simulink model "tqdtqr_rebuild_V3"  (R2021b)
settings: Solver=VariableStepAuto  StartTime=0.0  StopTime=10.0  RelTol=1e-3
undefined symbols (not defined in the file): ATQD_AfterTqMinGain_X_Deg, ATQD_APSCreepBaseTqD_X_kph, ATQD_APSCreepBaseTqD_Y_Deg, ATQD_APSCreepBaseTqR_X_kph, ATQD_APSCreepBaseTqR_Y_Deg, ATQD_APSCreepIterm_X_kph, ATQD_APSCreepIterm_Y_kph, ATQD_APSCreepPterm_X_kph, ATQD_APSCreepPterm_Y_kph, ATQD_APSDecReq_X_kph, ATQD_APSDecReq_Y_mps2, ATQD_APSDecReqCMD_X_kph, ATQD_APSDecReqTs_X_pct, ATQD_APSDecTimeGain_X_Deg, ATQD_APSDecTimeGain_Y_s, ATQD_APSReqLowSpd_X_Deg, ATQD_AutoHoldReleaseBPS_X_Deg, ATQD_AWDLoadTrqnsGain_X_kg, ATQD_AWDLoadTrqnsGain_Y_pct, ATQD_BOSEnBPSPosn_X_kph, ATQD_BOSMap_X_rpm, ATQD_BOSMap_Y_pct, ATQD_CreepBaseTqD_X_kph, ATQD_CreepBaseTqD_Y_Deg, ATQD_CreepBaseTqR_X_kph, ATQD_CreepBaseTqR_Y_Deg, ATQD_CreepBPSDisPosn_X_Deg, ATQD_CreepBPSDisPosnR_X_Deg, ATQD_CreepBPSEnPosn_X_Deg, ATQD_CreepBPSEnPosnR_X_Deg, ATQD_CreepDeltaTq_X_kph, ATQD_CreepIterm_X_kph, ATQD_CreepIterm_Y_kph, ATQD_CreepItermMaxLimit_X_pct, ATQD_CreepPreloadTime_X_kph, ATQD_CreepPreloadTq_X_kph, ATQD_CreepPreloadTq_Y_s, ATQD_CreepProtTq_X_Deg, ATQD_CreepPterm_X_kph, ATQD_CreepPterm_Y_kph, ATQD_CreepRrTqSpRat_X_rpm, ATQD_CreepRrTqSpRat_Y_Nm, ATQD_CreepTargetSpdD_X_pct, ATQD_CreepTargetSpdR_X_pct, ATQD_CreepUpLimitTq_X_rpm, ATQD_DecIneOPDHoldEnDelay_X_Deg, ATQD_DecIneOPDHoldEnDelay_Y_bar, ATQD_ECOTqMapD_X_rpm, ATQD_ECOTqMapD_Y_pct, ATQD_EMTqMapD_X_rpm, ATQD_EMTqMapD_Y_pct, ATQD_EOPDTqMapDCon_X_rpm, ATQD_EOPDTqMapDCon_Y_Deg, ATQD_EstInitVehWeight_X_c, ATQD_FAfterTqCMDGain_X_rpm, ATQD_FAfterTqCMDGain_Y_pct, ATQD_ForceLowSpd_X_Deg, ATQD_ForcePLimitSpd_X_Deg, ATQD_FrLossMAPLowV_X_rpm, ATQD_FrLossMAPLowV_Y_Nm ... (+949)
libraries: simulink x235, hcu_lib x208, tqr x63, tqd x6
(part 2 of 37)

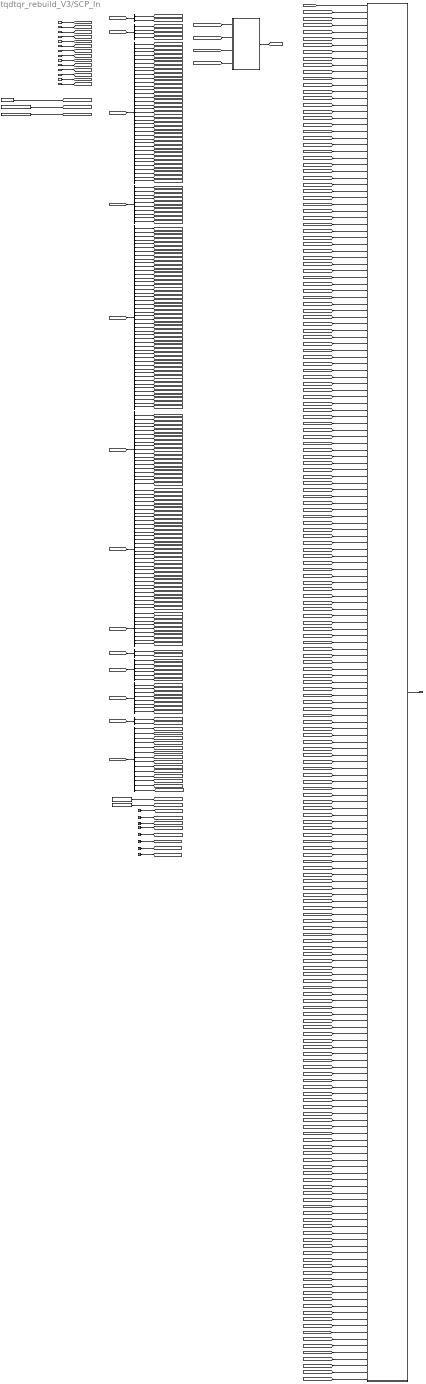
== system tqdtqr_rebuild_V3/SCP_In ==
  task_time_s : Inport
  BDHP_outputs : Inport  Port=2
  BPMM_outputs : Inport  Port=3
  BINP_CAN1_outputs : Inport  Port=4
  BINP_CAN2_outputs : Inport  Port=5
  BINP_CAN3_outputs : Inport  Port=6
  BINP_CAN4_outputs : Inport  Port=7
  BVMC_outputs : Inport  Port=8
  BINP_GPIO_outputs : Inport  Port=9
  BBCM_outputs : Inport  Port=10
  BINP_CAN6_outputs : Inport  Port=11
  BINP_SYS_outputs : Inport  Port=12
  BINP_APM_outputs : Inport  Port=13
  BDDM_outputs : Inport  Port=14
  Bus Selector : BusSelector  OutputSignals=VINP_IVIPWModeReq_enum,VINP_IVICreepSWReq_flg,VINP_RollModeSWCmd_enum,VINP_IVIPwrLockSW_enum,VINP_IVIISAOffsetSpd_enum,VINP_Distanceunit_flg,VINP_SmartEcoModeSW_flg,VINP_IVISnowModeCmd_flg,VINP_IVIACCAdaptiveSta_flg,VINP_IVITrailerModeSWSta_flg
  Bus Selector1 : BusSelector  OutputSignals=VDHP_ActAPSPosn_pct,VDHP_LowIdleAccPedal_flg
  Bus Selector10 : BusSelector  OutputSignals=VBCM_BrakeLamp_flg,VBCM_UserNow_enum
  Bus Selector11 : BusSelector  OutputSignals=VINP_FlashRegenMode_enum,VINP_VehicleType_enum,VINP_SWCType_enum,VINP_DIDGetDynoMode_flg,VINP_CAN1BusOff_flg,VINP_CAN1BusError_flg,VINP_CAN2BusOff_flg,VINP_CAN2BusError_flg
  Bus Selector12 : BusSelector  OutputSignals=VINP_CAASSta_enum,VINP_APSStaSystem_enum
  Bus Selector15 : BusSelector  OutputSignals=VDDM_VCURAPSErrLv2_flg,VDDM_VCURAPSErrLv3_flg,VDDM_EPBSigErrCFS_flg,VDDM_EPB1Err_flg,VDDM_ESC1Err_flg,VDDM_ESC5Err_flg,VDDM_LimpHomeAct_flg,VDDM_VehMalfunLevel_enum,VDDM_Shifter1Err_flg,VDDM_ShifterSigErrCFS_flg,VDDM_MCUF1Err_flg,VDDM_MCUR1Err_flg,VDDM_RegenErrCFS_flg,VDDM_4D2CErr_flg
  Bus Selector2 : BusSelector  OutputSignals=VINP_VehSpeed_kph,VINP_BrkSwSta_flg,VINP_BrkSwV_flg,VINP_BrkPedalPos_pct,VINP_BrkPedalPosSta_flg,VINP_FrPTCSActive_flg,VINP_RrPTCSActive_flg,VINP_FrntAxlTrqReqDrv_Nm,VINP_RearAxlTrqReqDrv_Nm,VINP_FrRBCActive_flg,VINP_RrRBCActive_flg,VINP_FrntAxlTrqReqBrk_Nm,VINP_RearAxlTrqReqBrk_Nm,VINP_CrashOutputSts_enum,VINP_LongAccel_Gps,VINP_EPBCarWashMode_flg,VINP_EPBErrSta_enum,VINP_EPBSta_enum,VINP_DOASta_flg,VINP_GRADE_Deg,VINP_HSAActive_flg,VINP_DriverSeatBeltCmd_flg,VINP_AVHActive_flg,VINP_PsngrSeatBeltCmd_flg,VINP_RDriverSeatBeltCmd_flg,VINP_RCenterSeatBeltCmd_flg,VINP_RPsngrSeatBeltCmd_flg,VINP_YawRate_degps,VINP_SASAngle_Deg,VINP_ESCActive_flg,VINP_ABSActive_flg,VINP_LFRawWhlSpeed_kph,VINP_LRRawWhlSpeed_kph,VINP_RFRawWhlSpeed_kph,VINP_RRRawWhlSpeed_kph,VINP_ESCOFFStatus_enum,VINP_MCPressure_bar
  Bus Selector3 : BusSelector  OutputSignals=VINP_BrakeSWGPIO_flg,VINP_CrashSignalGPIO_flg,VINP_DrDoorSW_flg,VINP_SeatSW_flg,VINP_HoodSW_flg,VINP_TailgateSW_flg,VINP_PsDoorSW_flg,VINP_RRDoorSW_flg,VINP_RLDoorSW_flg
  Bus Selector4 : BusSelector  OutputSignals=VINP_ShifterHandleCmd_enum,VINP_HVBPwrAvailDchrg_kW,VINP_HVBPwrAvailChrg_kW,VINP_HVBattErr_flg,VINP_DCDCFaultSta_enum,VINP_ChrgPlugSta_enum,VINP_HVBattSOC_pct,VINP_HVBattSOCDis_pct,VINP_HVBMTempMax_C,VINP_HVBMTempMin_C,VINP_ShifterFailsta_enum,VINP_CANMsgValidMCUNR1_flg,VINP_FrEDURotateDirctionNidec_enum,VINP_FrEDURotateDirction_enum,VINP_RrEDURotateDirctionNidec_enum,VINP_RrEDURotateDirction_enum,VINP_FrTMSpdNidec_rpm,VINP_FrTMSpd_rpm,VINP_RrTMSpdNidec_rpm,VINP_RrTMSpd_rpm,VINP_FrRegenAvailTqNidec_Nm,VINP_FrRegenAvailTq_Nm,VINP_RrRegenAvailTqNidec_Nm,VINP_RrRegenAvailTq_Nm,VINP_FrEDURealTMTqNidec_Nm,VINP_FrEDURealTMTq_Nm,VINP_RrEDURealTMTqNidec_Nm,VINP_RrEDURealTMTq_Nm,VINP_FrMotorAvailTqNidec_Nm,VINP_FrMotorAvailTq_Nm,VINP_RrMotorAvailTqNidec_Nm,VINP_RrMotorAvailTq_Nm,VINP_MCUWarnFNidec_enum,VINP_MCUWarnF_enum,VINP_MCUWarnRNidec_enum,VINP_MCUWarnR_enum,VINP_FrMCUDCBusVoltNidec_V,VINP_FrMCUDCBusVolt_V,VINP_RrMCUDCBusVoltNidec_V,VINP_RrMCUDCBusVolt_V,VINP_FrMCUTempNidec_C,VINP_FrMCUTemp_C,VINP_FrTMTempNidec_C,VINP_FrTMTemp_C,VINP_RrMCUTempNidec_C,VINP_RrMCUTemp_C,VINP_RrTMTempNidec_C,VINP_RrTMTemp_C
  Bus Selector5 : BusSelector  OutputSignals=VVMC_ADASForceIdle_flg,VVMC_ACCRequiredAccel_mps2,VVMC_ACCVehHoldReq_flg,VVMC_ADASActive_flg,VVMC_ADASWhlTqReq_Nm,VVMC_CruzActive_flg,VVMC_CruzWhlTqReq_Nm,VVMC_MSAActive_flg,VVMC_MSAWhlTqReq_Nm,VVMC_APSActive_flg,VVMC_APSSpeedCMD_kph,VVMC_APSShiftPosnReq_enum,VVMC_ACCPedalOvrd_flg,VVMC_LongAcc_Gps,VVMC_ActMaxSlideRate_pct,VVMC_EstSlope_Deg,VVMC_APSReq_enum,VVMC_RWDRDCActive_enum,VVMC_ActLRSlideRate_pct,VVMC_ActRRSlideRate_pct,VVMC_ActStESCYaw_Dps,VVMC_CCCtrlSta_enum,VVMC_MSACtrlSta_enum,VVMC_LVDAACCStatusInformation_flg,VVMC_ACCObjDist_m,VVMC_MeterIndSpeed_raw32,VVMC_RearTqRatio_rat,VVMC_CalibratedGyroY_Dps,VVMC_CAASActive_flg,VVMC_SetACCDisableAPS_flg,VVMC_CCPedalOvrd_flg,VVMC_MSAWhlTqActive_flg
  Bus Selector6 : BusSelector  OutputSignals=VINP_SWCResUpSta_flg,VINP_SWCSetdownSta_flg,VINP_SWCACCSta_flg,VINP_SWCCANCELSta_flg,VINP_SWC2LScrollUpSta_flg,VINP_SWC2LScrollDownSta_flg,VINP_SWC2LScrollPressSta_flg,VINP_SWC2LADASSta_flg,VINP_SWC2RScrollPressSta_flg,VINP_SWC2RScrollUpSta_flg,VINP_SWC2RScrollDownSta_flg,VINP_SWC2LDriveModeSta_flg,VINP_SWC2RRightSta_flg,VINP_SWC2RLeftSta_flg,VINP_SWC2RCustomizeSta_flg,VINP_SWC2LRegenUpSta_flg,VINP_SWC2RRegenDownSta_flg,VINP_SWCRegenDown_flg,VINP_SWCRegenUp_flg
  Bus Selector7 : BusSelector  OutputSignals=VPMM_PowerSta_enum,VPMM_DrivetrainSelect_enum,VPMM_SysPowerMode_enum,VPMM_DrSeatSta_enum
  Bus Selector9 : BusSelector  OutputSignals=VINP_ADASISASta_enum,VINP_ADASVehSpdLim_enum,VINP_ADASACCSta_enum,VINP_ADASSLIFSpdLim_enum,VINP_ADASAEBSta_enum,VINP_ACCVehHoldReq_flg
  Constant : Constant  Value=ZERO_INT
  Constant1 : Constant  Value=KTQD_BCMUserNowSetting_enum
  Constant12 : Constant  Value=KTQD_DIDNVHPedalLim_flg
  Constant2 : Constant  Value=KTQD_IVIRockModeCmd_flg
  Constant3 : Constant  Value=KTQD_DIDExhibitMode_enum
  Ground{,1..7} (8 alike) : Ground
  Input Signal : Subsystem
  Invalid Condition : Subsystem
  BSCPIn_outputs : Outport
  wires:
  task_time_s/1 -> [task_time_s]
  BDHP_outputs/1 -> [BDHP_outputs]
  BPMM_outputs/1 -> [BPMM_outputs]
  BINP_CAN1_outputs/1 -> [BINP_CAN1_outputs]
  BINP_CAN2_outputs/1 -> [BINP_CAN2_outputs]
  BINP_CAN3_outputs/1 -> [BINP_CAN3_outputs]
  BINP_CAN4_outputs/1 -> [BINP_CAN4_outputs]
  BVMC_outputs/1 -> [BVMC_outputs]
  BINP_GPIO_outputs/1 -> [BINP_GPIO_outputs]
  BBCM_outputs/1 -> [BBCM_outputs]
  BINP_CAN6_outputs/1 -> [BINP_CAN6_outputs]
  BINP_SYS_outputs/1 -> [BINP_SYS_outputs]
  BINP_APM_outputs/1 -> [BINP_APM_outputs]
  BDDM_outputs/1 -> [BDDM_outputs]
  [BDHP_outputs] -> Bus Selector1/1
  Bus Selector1/1 -> [VDHP_ActAPSPosn_pct]  "<VDHP_ActAPSPosn_pct>"
  Bus Selector1/2 -> [VDHP_LowIdleAccPedal_flg]  "<VDHP_LowIdleAccPedal_flg>"
  [BPMM_outputs] -> Bus Selector7/1
  Bus Selector7/1 -> [VPMM_PowerSta_enum]  "<VPMM_PowerSta_enum>"
  Bus Selector7/2 -> [VPMM_DrivetrainSelect_enum]  "<VPMM_DrivetrainSelect_enum>"
  Bus Selector7/3 -> [VPMM_SysPowerMode_enum]  "<VPMM_SysPowerMode_enum>"
  [BINP_CAN1_outputs] -> Bus Selector2/1
  Bus Selector2/1 -> [VINP_VehSpeed_kph]  "<VINP_VehSpeed_kph>"
  Bus Selector2/2 -> [VINP_BrkSwSta_flg]  "<VINP_BrkSwSta_flg>"
  Bus Selector2/3 -> [VINP_BrkSwV_flg]  "<VINP_BrkSwV_flg>"
  Bus Selector2/4 -> [VINP_BrkPedalPos_pct]  "<VINP_BrkPedalPos_pct>"
  Bus Selector2/5 -> [VINP_BrkPedalPosSta_flg]  "<VINP_BrkPedalPosSta_flg>"
  Bus Selector2/6 -> [VINP_FrPTCSActive_flg]  "<VINP_FrPTCSActive_flg>"
  Bus Selector2/7 -> [VINP_RrPTCSActive_flg]  "<VINP_RrPTCSActive_flg>"
  Bus Selector2/8 -> [VINP_FrntAxlTrqReqDrv_Nm]  "<VINP_FrntAxlTrqReqDrv_Nm>"
  Bus Selector2/9 -> [VINP_RearAxlTrqReqDrv_Nm]  "<VINP_RearAxlTrqReqDrv_Nm>"
  Bus Selector2/10 -> [VINP_FrRBCActive_flg]  "<VINP_FrRBCActive_flg>"
  Bus Selector2/11 -> [VINP_RrRBCActive_flg]  "<VINP_RrRBCActive_flg>"
  Bus Selector2/12 -> [VINP_FrntAxlTrqReqBrk_Nm]  "<VINP_FrntAxlTrqReqBrk_Nm>"
  Bus Selector2/13 -> [VINP_RearAxlTrqReqBrk_Nm]  "<VINP_RearAxlTrqReqBrk_Nm>"
  Bus Selector2/14 -> [VINP_CrashOutputSts_enum]  "<VINP_CrashOutputSts_enum>"
  Bus Selector2/15 -> [VINP_LongAccel_Gps]  "<VINP_LongAccel_Gps>"
  Bus Selector2/16 -> [VINP_EPBCarWashMode_flg]  "<VINP_EPBCarWashMode_flg>"
  Bus Selector2/17 -> [VINP_EPBErrSta_enum]  "<VINP_EPBErrSta_enum>"
  Bus Selector2/18 -> [VINP_EPBSta_enum]  "<VINP_EPBSta_enum>"
  Bus Selector2/19 -> [VINP_DOASta_flg]  "<VINP_DOASta_flg>"
  Bus Selector2/20 -> [VINP_GRADE_Deg]  "<VINP_GRADE_Deg>"
  Bus Selector2/21 -> [VINP_HSAActive_flg]  "<VINP_HSAActive_flg>"
  Bus Selector2/22 -> [VINP_DriverSeatBeltCmd_flg]  "<VINP_DriverSeatBeltCmd_flg>"
  Bus Selector2/23 -> [VINP_AVHActive_flg]  "<VINP_AVHActive_flg>"
  Bus Selector2/24 -> [VINP_PsngrSeatBeltCmd_flg]  "<VINP_PsngrSeatBeltCmd_flg>"
  Bus Selector2/25 -> [VINP_RDriverSeatBeltCmd_flg]  "<VINP_RDriverSeatBeltCmd_flg>"
  Bus Selector2/26 -> [VINP_RCenterSeatBeltCmd_flg]  "<VINP_RCenterSeatBeltCmd_flg>"
  Bus Selector2/27 -> [VINP_RPsngrSeatBeltCmd_flg]  "<VINP_RPsngrSeatBeltCmd_flg>"
  Bus Selector2/28 -> [VINP_YawRate_degps]  "<VINP_YawRate_degps>"
  Bus Selector2/29 -> [VINP_SASAngle_Deg]  "<VINP_SASAngle_Deg>"
  Bus Selector2/30 -> [VINP_ESCActive_flg]  "<VINP_ESCActive_flg>"
  Bus Selector2/31 -> [VINP_ABSActive_flg]  "<VINP_ABSActive_flg>"
  Bus Selector2/32 -> [VINP_LFRawWhlSpeed_kph]  "<VINP_LFRawWhlSpeed_kph>"
  Bus Selector2/33 -> [VINP_LRRawWhlSpeed_kph]  "<VINP_LRRawWhlSpeed_kph>"
  Bus Selector2/34 -> [VINP_RFRawWhlSpeed_kph]  "<VINP_RFRawWhlSpeed_kph>"
  Bus Selector2/35 -> [VINP_RRRawWhlSpeed_kph]  "<VINP_RRRawWhlSpeed_kph>"
  Bus Selector2/36 -> [VINP_ESCOFFStatus_enum]  "<VINP_ESCOFFStatus_enum>"
  [BINP_CAN2_outputs] -> Bus Selector/1
  Bus Selector/1 -> [VINP_IVIPWModeReq_enum]  "<VINP_IVIPWModeReq_enum>"
  Bus Selector/2 -> [VINP_IVICreepSWReq_flg]  "<VINP_IVICreepSWReq_flg>"
  Bus Selector/3 -> [VINP_RollModeSWCmd_enum]  "<VINP_RollModeSWCmd_enum>"
  Bus Selector/4 -> [VINP_IVIPwrLockSW_enum]  "<VINP_IVIPwrLockSW_enum>"
  Bus Selector/5 -> [VINP_IVIISAOffsetSpd_enum]  "<VINP_IVIISAOffsetSpd_enum>"
  Bus Selector/6 -> [VINP_Distanceunit_flg]  "<VINP_Distanceunit_flg>"
  Bus Selector/7 -> [VINP_SmartEcoModeSW_flg]  "<VINP_SmartEcoModeSW_flg>"
  Bus Selector/8 -> [VINP_IVISnowModeCmd_flg]  "<VINP_IVISnowModeCmd_flg>"
  Bus Selector/9 -> [VINP_IVIACCAdaptiveSta_flg]  "<VINP_IVIACCAdaptiveSta_flg>"
  Bus Selector/10 -> [VINP_IVITrailerModeSWSta_flg]  "<VINP_IVITrailerModeSWSta_flg>"
  [BINP_CAN3_outputs] -> Bus Selector4/1
  Bus Selector4/1 -> [VINP_ShifterHandleCmd_enum]  "<VINP_ShifterHandleCmd_enum>"
  Bus Selector4/2 -> [VINP_HVBPwrAvailDchrg_kW]  "<VINP_HVBPwrAvailDchrg_kW>"
  Bus Selector4/3 -> [VINP_HVBPwrAvailChrg_kW]  "<VINP_HVBPwrAvailChrg_kW>"
  Bus Selector4/4 -> [VINP_HVBattErr_flg]  "<VINP_HVBattErr_flg>"
  Bus Selector4/5 -> [VINP_DCDCFaultSta_enum]  "<VINP_DCDCFaultSta_enum>"
  Bus Selector4/6 -> [VINP_ChrgPlugSta_enum]  "<VINP_ChrgPlugSta_enum>"
  Bus Selector4/7 -> [VINP_HVBattSOC_pct]  "<VINP_HVBattSOC_pct>"
  Bus Selector4/8 -> [VINP_HVBattSOCDis_pct]  "<VINP_HVBattSOCDis_pct>"
  Bus Selector4/9 -> [VINP_HVBMTempMax_C]  "<VINP_HVBMTempMax_C>"
  Bus Selector4/10 -> [VINP_HVBMTempMin_C]  "<VINP_HVBMTempMin_C>"
  Bus Selector4/11 -> [VINP_ShifterFailsta_enum]  "<VINP_ShifterFailsta_enum>"
  Bus Selector4/12 -> [VINP_CANMsgValidMCUNR1_flg]  "<VINP_CANMsgValidMCUNR1_flg>"
  Bus Selector4/13 -> [VINP_FrEDURotateDirctionNidec_enum]  "<VINP_FrEDURotateDirctionNidec_enum>"
  Bus Selector4/14 -> [VINP_FrEDURotateDirction_enum]  "<VINP_FrEDURotateDirction_enum>"
  Bus Selector4/15 -> [VINP_RrEDURotateDirctionNidec_enum]  "<VINP_RrEDURotateDirctionNidec_enum>"
  Bus Selector4/16 -> [VINP_RrEDURotateDirction_enum]  "<VINP_RrEDURotateDirction_enum>"
  Bus Selector4/17 -> [VINP_FrTMSpdNidec_rpm]  "<VINP_FrTMSpdNidec_rpm>"
  Bus Selector4/18 -> [VINP_FrTMSpd_rpm]  "<VINP_FrTMSpd_rpm>"
  Bus Selector4/19 -> [VINP_RrTMSpdNidec_rpm]  "<VINP_RrTMSpdNidec_rpm>"
  Bus Selector4/20 -> [VINP_RrTMSpd_rpm]  "<VINP_RrTMSpd_rpm>"
  Bus Selector4/21 -> [VINP_FrRegenAvailTqNidec_Nm]  "<VINP_FrRegenAvailTqNidec_Nm>"
  Bus Selector4/22 -> [VINP_FrRegenAvailTq_Nm]  "<VINP_FrRegenAvailTq_Nm>"
  Bus Selector4/23 -> [VINP_RrRegenAvailTqNidec_Nm]  "<VINP_RrRegenAvailTqNidec_Nm>"
  Bus Selector4/24 -> [VINP_RrRegenAvailTq_Nm]  "<VINP_RrRegenAvailTq_Nm>"
  Bus Selector4/25 -> [VINP_FrEDURealTMTqNidec_Nm]  "<VINP_FrEDURealTMTqNidec_Nm>"
  Bus Selector4/26 -> [VINP_FrEDURealTMTq_Nm]  "<VINP_FrEDURealTMTq_Nm>"
  Bus Selector4/27 -> [VINP_RrEDURealTMTqNidec_Nm]  "<VINP_RrEDURealTMTqNidec_Nm>"
  Bus Selector4/28 -> [VINP_RrEDURealTMTq_Nm]  "<VINP_RrEDURealTMTq_Nm>"
  Bus Selector4/29 -> [VINP_FrMotorAvailTqNidec_Nm]  "<VINP_FrMotorAvailTqNidec_Nm>"
  Bus Selector4/30 -> [VINP_FrMotorAvailTq_Nm]  "<VINP_FrMotorAvailTq_Nm>"
  Bus Selector4/31 -> [VINP_RrMotorAvailTqNidec_Nm]  "<VINP_RrMotorAvailTqNidec_Nm>"
  Bus Selector4/32 -> [VINP_RrMotorAvailTq_Nm]  "<VINP_RrMotorAvailTq_Nm>"
  Bus Selector4/33 -> [VINP_MCUWarnFNidec_enum]  "<VINP_MCUWarnFNidec_enum>"
  Bus Selector4/34 -> [VINP_MCUWarnF_enum]  "<VINP_MCUWarnF_enum>"
  Bus Selector4/35 -> [VINP_MCUWarnRNidec_enum]  "<VINP_MCUWarnRNidec_enum>"
  Bus Selector4/36 -> [VINP_MCUWarnR_enum]  "<VINP_MCUWarnR_enum>"
  Bus Selector4/37 -> [VINP_FrMCUDCBusVoltNidec_V]  "<VINP_FrMCUDCBusVoltNidec_V>"
  Bus Selector4/38 -> [VINP_FrMCUDCBusVolt_V]  "<VINP_FrMCUDCBusVolt_V>"
  Bus Selector4/39 -> [VINP_RrMCUDCBusVoltNidec_V]  "<VINP_RrMCUDCBusVoltNidec_V>"
  Bus Selector4/40 -> [VINP_RrMCUDCBusVolt_V]  "<VINP_RrMCUDCBusVolt_V>"
  Bus Selector4/41 -> [VINP_FrMCUTempNidec_C]  "<VINP_FrMCUTempNidec_C>"
  Bus Selector4/42 -> [VINP_FrMCUTemp_C]  "<VINP_FrMCUTemp_C>"
  Bus Selector4/43 -> [VINP_FrTMTempNidec_C]  "<VINP_FrTMTempNidec_C>"
  Bus Selector4/44 -> [VINP_FrTMTemp_C]  "<VINP_FrTMTemp_C>"
  Bus Selector4/45 -> [VINP_RrMCUTempNidec_C]  "<VINP_RrMCUTempNidec_C>"
  Bus Selector4/46 -> [VINP_RrMCUTemp_C]  "<VINP_RrMCUTemp_C>"
  Bus Selector4/47 -> [VINP_RrTMTempNidec_C]  "<VINP_RrTMTempNidec_C>"
  Bus Selector4/48 -> [VINP_RrTMTemp_C]  "<VINP_RrTMTemp_C>"
  [BINP_CAN4_outputs] -> Bus Selector6/1
  Bus Selector6/1 -> [VINP_SWCResUpSta_flg]  "<VINP_SWCResUpSta_flg>"
  Bus Selector6/2 -> [VINP_SWCSetdownSta_flg]  "<VINP_SWCSetdownSta_flg>"
  Bus Selector6/3 -> [VINP_SWCACCSta_flg]  "<VINP_SWCACCSta_flg>"
  Bus Selector6/4 -> [VINP_SWCCANCELSta_flg]  "<VINP_SWCCANCELSta_flg>"
  Bus Selector6/5 -> [VINP_SWC2LScrollUpSta_flg]  "<VINP_SWC2LScrollUpSta_flg>"
  Bus Selector6/6 -> [VINP_SWC2LScrollDownSta_flg]  "<VINP_SWC2LScrollDownSta_flg>"
  Bus Selector6/7 -> [VINP_SWC2LScrollPressSta_flg]  "<VINP_SWC2LScrollPressSta_flg>"
  Bus Selector6/8 -> [VINP_SWC2LADASSta_flg]  "<VINP_SWC2LADASSta_flg>"
  Bus Selector6/9 -> [VINP_SWC2RScrollPressSta_flg]  "<VINP_SWC2RScrollPressSta_flg>"
  Bus Selector6/10 -> [VINP_SWC2RScrollUpSta_flg]  "<VINP_SWC2RScrollUpSta_flg>"
  Bus Selector6/11 -> [VINP_SWC2RScrollDownSta_flg]  "<VINP_SWC2RScrollDownSta_flg>"
  Bus Selector6/12 -> [VINP_SWC2LDriveModeSta_flg]  "<VINP_SWC2LDriveModeSta_flg>"
  Bus Selector6/13 -> [VINP_SWC2RRightSta_flg]  "<VINP_SWC2RRightSta_flg>"
  Bus Selector6/14 -> [VINP_SWC2RLeftSta_flg]  "<VINP_SWC2RLeftSta_flg>"
  Bus Selector6/15 -> [VINP_SWC2RCustomizeSta_flg]  "<VINP_SWC2RCustomizeSta_flg>"
  Bus Selector6/16 -> [VINP_SWC2LRegenUpSta_flg]  "<VINP_SWC2LRegenUpSta_flg>"
  Bus Selector6/17 -> [VINP_SWC2RRegenDownSta_flg]  "<VINP_SWC2RRegenDownSta_flg>"
  Bus Selector6/18 -> [VINP_SWCRegenDown_flg]  "<VINP_SWCRegenDown_flg>"
  Bus Selector6/19 -> [VINP_SWCRegenUp_flg]  "<VINP_SWCRegenUp_flg>"
  [BVMC_outputs] -> Bus Selector5/1
  Bus Selector5/1 -> [VVMC_ADASForceIdle_flg]  "<VVMC_ADASForceIdle_flg>"
  Bus Selector5/2 -> [VVMC_ACCRequiredAccel_mps2]  "<VVMC_ACCRequiredAccel_mps2>"
  Bus Selector5/3 -> [VVMC_ACCVehHoldReq_flg]  "<VVMC_ACCVehHoldReq_flg>"
  Bus Selector5/4 -> [VVMC_ADASActive_flg]  "<VVMC_ADASActive_flg>"
  Bus Selector5/5 -> [VVMC_ADASWhlTqReq_Nm]  "<VVMC_ADASWhlTqReq_Nm>"
  Bus Selector5/6 -> [VVMC_CruzActive_flg]  "<VVMC_CruzActive_flg>"
  Bus Selector5/7 -> [VVMC_CruzWhlTqReq_Nm]  "<VVMC_CruzWhlTqReq_Nm>"
  Bus Selector5/8 -> [VVMC_MSAActive_flg]  "<VVMC_MSAActive_flg>"
  Bus Selector5/9 -> [VVMC_MSAWhlTqReq_Nm]  "<VVMC_MSAWhlTqReq_Nm>"
  Bus Selector5/10 -> [VVMC_APSActive_flg]  "<VVMC_APSActive_flg>"
  Bus Selector5/11 -> [VVMC_APSSpeedCMD_kph]  "<VVMC_APSSpeedCMD_kph>"
  Bus Selector5/12 -> [VVMC_APSShiftPosnReq_enum]  "<VVMC_APSShiftPosnReq_enum>"
  Bus Selector5/13 -> [VVMC_ACCPedalOvrd_flg]  "<VVMC_ACCPedalOvrd_flg>"
  Bus Selector5/14 -> [VVMC_LongAcc_Gps]  "<VVMC_LongAcc_Gps>"
  Bus Selector5/15 -> [VVMC_ActMaxSlideRate_pct]  "<VVMC_ActMaxSlideRate_pct>"
  Bus Selector5/16 -> [VVMC_EstSlope_Deg]  "<VVMC_EstSlope_Deg>"
  Bus Selector5/17 -> [VVMC_APSReq_enum]  "<VVMC_APSReq_enum>"
  Bus Selector5/18 -> [VVMC_RWDRDCActive_enum]  "<VVMC_RWDRDCActive_enum>"
  Bus Selector5/19 -> [VVMC_ActLRSlideRate_pct]  "<VVMC_ActLRSlideRate_pct>"
  Bus Selector5/20 -> [VVMC_ActRRSlideRate_pct]  "<VVMC_ActRRSlideRate_pct>"
  Bus Selector5/21 -> [VVMC_ActStESCYaw_Dps]  "<VVMC_ActStESCYaw_Dps>"
  Bus Selector5/22 -> [VVMC_CCCtrlSta_enum]  "<VVMC_CCCtrlSta_enum>"
  Bus Selector5/23 -> [VVMC_MSACtrlSta_enum]  "<VVMC_MSACtrlSta_enum>"
  Bus Selector5/24 -> [VVMC_LVDAACCStatusInformation_flg]  "<VVMC_LVDAACCStatusInformation_flg>"
  Bus Selector5/25 -> [VVMC_ACCObjDist_m]  "<VVMC_ACCObjDist_m>"
  Bus Selector5/26 -> [VVMC_MeterIndSpeed_raw32]  "<VVMC_MeterIndSpeed_raw32>"
  Bus Selector5/27 -> [VVMC_RearTqRatio_rat]  "<VVMC_RearTqRatio_rat>"
  Bus Selector5/28 -> [VVMC_CalibratedGyroY_Dps]  "<VVMC_CalibratedGyroY_Dps>"
  Bus Selector5/29 -> [VVMC_CAASActive_flg]  "<VVMC_CAASActive_flg>"
  Bus Selector5/30 -> [VVMC_SetACCDisableAPS_flg]  "<VVMC_SetACCDisableAPS_flg>"
  [BINP_GPIO_outputs] -> Bus Selector3/1
  Bus Selector3/1 -> [VINP_BrakeSWGPIO_flg]  "<VINP_BrakeSWGPIO_flg>"
  Bus Selector3/2 -> [VINP_CrashSignalGPIO_flg]  "<VINP_CrashSignalGPIO_flg>"
  Bus Selector3/3 -> [VINP_DrDoorSW_flg]  "<VINP_DrDoorSW_flg>"
  Bus Selector3/4 -> [VINP_SeatSW_flg]  "<VINP_SeatSW_flg>"
  Bus Selector3/5 -> [VINP_HoodSW_flg]  "<VINP_HoodSW_flg>"
  Bus Selector3/6 -> [VINP_TailgateSW_flg]  "<VINP_TailgateSW_flg>"
  Bus Selector3/7 -> [VINP_PsDoorSW_flg]  "<VINP_PsDoorSW_flg>"
  Bus Selector3/8 -> [VINP_RRDoorSW_flg]  "<VINP_RRDoorSW_flg>"
  Bus Selector3/9 -> [VINP_RLDoorSW_flg]  "<VINP_RLDoorSW_flg>"
  [BBCM_outputs] -> Bus Selector10/1
  Bus Selector10/1 -> [VBCM_BrakeLamp_flg]  "<VBCM_BrakeLamp_flg>"
  Bus Selector10/2 -> [VBCM_UserNow_enum]  "<VBCM_UserNow_enum>"
  [BINP_CAN6_outputs] -> Bus Selector9/1
  Bus Selector9/1 -> [VINP_ADASISASta_enum]  "<VINP_ADASISASta_enum>"
  Bus Selector9/2 -> [VINP_ADASVehSpdLim_enum]  "<VINP_ADASVehSpdLim_enum>"
  Bus Selector9/3 -> [VINP_ADASACCSta_enum]  "<VINP_ADASACCSta_enum>"
  Bus Selector9/4 -> [VINP_ADASSLIFSpdLim_enum]  "<VINP_ADASSLIFSpdLim_enum>"
  Bus Selector9/5 -> [VINP_ADASAEBSta_enum]  "<VINP_ADASAEBSta_enum>"
  [BINP_SYS_outputs] -> Bus Selector11/1
  Bus Selector11/1 -> [VINP_FlashRegenMode_enum]  "<VINP_FlashRegenMode_enum>"
  Bus Selector11/2 -> [VINP_VehicleType_enum]  "<VINP_VehicleType_enum>"
  Bus Selector11/3 -> [VINP_SWCType_enum]  "<VINP_SWCType_enum>"
  [BINP_APM_outputs] -> Bus Selector12/1
  Bus Selector12/1 -> [VINP_CAASSta_enum]  "<VINP_CAASSta_enum>"
  Bus Selector12/2 -> [VINP_APSStaSystem_enum]  "<VINP_APSStaSystem_enum>"
  [BDDM_outputs] -> Bus Selector15/1
  Bus Selector15/1 -> [VDDM_VCURAPSErrLv2_flg]  "<VDDM_VCURAPSErrLv2_flg>"
  Bus Selector15/2 -> [VDDM_VCURAPSErrLv3_flg]  "<VDDM_VCURAPSErrLv3_flg>"
  Bus Selector15/3 -> [VDDM_EPBSigErrCFS_flg]  "<VDDM_EPBSigErrCFS_flg>"
  Bus Selector15/4 -> [VDDM_EPB1Err_flg]  "<VDDM_EPB1Err_flg>"
  Bus Selector15/5 -> [VDDM_ESC1Err_flg]  "<VDDM_ESC1Err_flg>"
  Bus Selector15/6 -> [VDDM_ESC5Err_flg]  "<VDDM_ESC5Err_flg>"
  Bus Selector15/7 -> [VDDM_LimpHomeAct_flg]  "<VDDM_LimpHomeAct_flg>"
  Bus Selector15/8 -> [VDDM_VehMalfunLevel_enum]  "<VDDM_VehMalfunLevel_enum>"
  Bus Selector15/9 -> [VDDM_Shifter1Err_flg]  "<VDDM_Shifter1Err_flg>"
  Bus Selector15/10 -> [VDDM_ShifterSigErrCFS_flg]  "<VDDM_ShifterSigErrCFS_flg>"
  Bus Selector15/11 -> [VDDM_MCUF1Err_flg]  "<VDDM_MCUF1Err_flg>"
  Bus Selector15/12 -> [VDDM_MCUR1Err_flg]  "<VDDM_MCUR1Err_flg>"
  Bus Selector15/13 -> [VDDM_RegenErrCFS_flg]  "<VDDM_RegenErrCFS_flg>"
  Bus Selector15/14 -> [VDDM_4D2CErr_flg]  "<VDDM_4D2CErr_flg>"
  Constant/1 -> [VINP_PBWMotorPos_enum]  "VINP_PBWMotorPos_enum"
  Constant2/1 -> [VINP_IVIEscapeModeCmd_flg]  "VTQD_IVIRockModeCmd_flg"
  Constant1/1 -> [VBCM_RegenModeUserSetting_enum]  "VTQD_BCMUserNowSetting_enum"
  [task_time_s] -> Input Signal/2(task_time_s)
  [VDHP_ActAPSPosn_pct] -> Input Signal/3(VDHP_ActAPSPosn_pct)
  [VDHP_LowIdleAccPedal_flg] -> Input Signal/4(VDHP_LowIdleAccPedal_flg)
  [VPMM_PowerSta_enum] -> Input Signal/5(VPMM_PowerSta_enum)
  [VPMM_DrivetrainSelect_enum] -> Input Signal/6(VPMM_DrivetrainSelect_enum)
  [VPMM_SysPowerMode_enum] -> Input Signal/7(VPMM_SysPowerMode_enum)
  [VINP_VehSpeed_kph] -> Input Signal/9(VINP_VehSpeed_kph)
  [VINP_BrkPedalPos_pct] -> Input Signal/12(VINP_BrkPedalPos_pct)
  [VINP_BrkPedalPosSta_flg] -> Input Signal/13(VINP_BrkPedalPosSta_flg)
  [VINP_FrPTCSActive_flg] -> Input Signal/14(VINP_FrPTCSActive_flg)
  [VINP_RrPTCSActive_flg] -> Input Signal/15(VINP_RrPTCSActive_flg)
  [VINP_FrntAxlTrqReqDrv_Nm] -> Input Signal/16(VINP_FrntAxlTrqReqDrv_Nm)
  [VINP_RearAxlTrqReqDrv_Nm] -> Input Signal/17(VINP_RearAxlTrqReqDrv_Nm)
  [VINP_FrRBCActive_flg] -> Input Signal/18(VINP_FrRBCActive_flg)
  [VINP_RrRBCActive_flg] -> Input Signal/19(VINP_RrRBCActive_flg)
  [VINP_FrntAxlTrqReqBrk_Nm] -> Input Signal/20(VINP_FrntAxlTrqReqBrk_Nm)
  [VINP_RearAxlTrqReqBrk_Nm] -> Input Signal/21(VINP_RearAxlTrqReqBrk_Nm)
  [VINP_CrashOutputSts_enum] -> Input Signal/22(VINP_CrashOutputSts_enum)
  [VINP_LongAccel_Gps] -> Input Signal/23(VINP_LongAccel_Gps)
  [VINP_EPBCarWashMode_flg] -> Input Signal/24(VINP_EPBCarWashMode_flg)
  [VINP_EPBErrSta_enum] -> Input Signal/25(VINP_EPBErrSta_enum)
  [VINP_EPBSta_enum] -> Input Signal/26(VINP_EPBSta_enum)
  [VINP_DOASta_flg] -> Input Signal/27(VINP_DOASta_flg)
  [VINP_GRADE_Deg] -> Input Signal/28(VINP_GRADE_Deg)
  [VINP_HSAActive_flg] -> Input Signal/29(VINP_HSAActive_flg)
  [VINP_DriverSeatBeltCmd_flg] -> Input Signal/30(VINP_DriverSeatBeltCmd_flg)
  [VINP_AVHActive_flg] -> Input Signal/31(VINP_AVHActive_flg)
  [VINP_PsngrSeatBeltCmd_flg] -> Input Signal/32(VINP_PsngrSeatBeltCmd_flg)
  [VINP_RDriverSeatBeltCmd_flg] -> Input Signal/33(VINP_RDriverSeatBeltCmd_flg)
  [VINP_RCenterSeatBeltCmd_flg] -> Input Signal/34(VINP_RCenterSeatBeltCmd_flg)
  [VINP_RPsngrSeatBeltCmd_flg] -> Input Signal/35(VINP_RPsngrSeatBeltCmd_flg)
  [VINP_YawRate_degps] -> Input Signal/36(VINP_YawRate_degps)
  [VINP_SASAngle_Deg] -> Input Signal/37(VINP_SASAngle_Deg)
  [VINP_ESCActive_flg] -> Input Signal/38(VINP_ESCActive_flg)
  [VINP_ABSActive_flg] -> Input Signal/39(VINP_ABSActive_flg)
  [VINP_LFRawWhlSpeed_kph] -> Input Signal/40(VINP_LFRawWhlSpeed_kph)
  [VINP_LRRawWhlSpeed_kph] -> Input Signal/41(VINP_LRRawWhlSpeed_kph)
  [VINP_RFRawWhlSpeed_kph] -> Input Signal/42(VINP_RFRawWhlSpeed_kph)
  [VINP_RRRawWhlSpeed_kph] -> Input Signal/43(VINP_RRRawWhlSpeed_kph)
  [VINP_ESCOFFStatus_enum] -> Input Signal/44(VINP_ESCOFFStatus_enum)
  [VINP_IVIPWModeReq_enum] -> Input Signal/46(VINP_IVIPWModeReq_enum)
  [VINP_IVICreepSWReq_flg] -> Input Signal/47(VINP_IVICreepSWReq_flg)
  [VINP_RollModeSWCmd_enum] -> Input Signal/48(VINP_RollModeSWCmd_enum)
  [VINP_IVIPwrLockSW_enum] -> Input Signal/49(VINP_IVIPwrLockSW_enum)
  [VINP_IVIISAOffsetSpd_enum] -> Input Signal/50(VINP_IVIISAOffsetSpd_enum)
  [VINP_Distanceunit_flg] -> Input Signal/51(VINP_Distanceunit_flg)
  [VINP_SmartEcoModeSW_flg] -> Input Signal/52(VINP_SmartEcoModeSW_flg)
  [VINP_IVISnowModeCmd_flg] -> Input Signal/53(VINP_IVISnowModeCmd_flg)
  [VINP_IVIACCAdaptiveSta_flg] -> Input Signal/54(VINP_IVIACCAdaptiveSta_flg)
  [VINP_IVITrailerModeSWSta_flg] -> Input Signal/55(VINP_IVITrailerModeSWSta_flg)
  [VINP_ShifterHandleCmd_enum] -> Input Signal/56(VINP_ShifterHandleCmd_enum)
  [VINP_HVBPwrAvailDchrg_kW] -> Input Signal/57(VINP_HVBPwrAvailDchrg_kW)
  [VINP_HVBPwrAvailChrg_kW] -> Input Signal/58(VINP_HVBPwrAvailChrg_kW)
  [VINP_HVBattErr_flg] -> Input Signal/59(VINP_HVBattErr_flg)
  [VINP_DCDCFaultSta_enum] -> Input Signal/60(VINP_DCDCFaultSta_enum)
  [VINP_ChrgPlugSta_enum] -> Input Signal/61(VINP_ChrgPlugSta_enum)
  [VINP_HVBattSOC_pct] -> Input Signal/62(VINP_HVBattSOC_pct)
  [VINP_HVBattSOCDis_pct] -> Input Signal/63(VINP_HVBattSOCDis_pct)
  [VINP_HVBMTempMax_C] -> Input Signal/64(VINP_HVBMTempMax_C)
  [VINP_HVBMTempMin_C] -> Input Signal/65(VINP_HVBMTempMin_C)
  [VINP_ShifterFailsta_enum] -> Input Signal/66(VINP_ShifterFailsta_enum)
  [VINP_CANMsgValidMCUNR1_flg] -> Input Signal/67(VINP_CANMsgValidMCUNR1_flg)
  [VINP_FrEDURotateDirctionNidec_enum] -> Input Signal/68(VINP_FrEDURotateDirctionNidec_enum)
  [VINP_FrEDURotateDirction_enum] -> Input Signal/69(VINP_FrEDURotateDirction_enum)
  [VINP_RrEDURotateDirctionNidec_enum] -> Input Signal/70(VINP_RrEDURotateDirctionNidec_enum)
  [VINP_RrEDURotateDirction_enum] -> Input Signal/71(VINP_RrEDURotateDirction_enum)
  [VINP_FrTMSpdNidec_rpm] -> Input Signal/72(VINP_FrTMSpdNidec_rpm)
  [VINP_FrTMSpd_rpm] -> Input Signal/73(VINP_FrTMSpd_rpm)
  [VINP_RrTMSpdNidec_rpm] -> Input Signal/74(VINP_RrTMSpdNidec_rpm)
  [VINP_RrTMSpd_rpm] -> Input Signal/75(VINP_RrTMSpd_rpm)
  [VINP_FrRegenAvailTqNidec_Nm] -> Input Signal/76(VINP_FrRegenAvailTqNidec_Nm)
  [VINP_FrRegenAvailTq_Nm] -> Input Signal/77(VINP_FrRegenAvailTq_Nm)
  [VINP_RrRegenAvailTqNidec_Nm] -> Input Signal/78(VINP_RrRegenAvailTqNidec_Nm)
  [VINP_RrRegenAvailTq_Nm] -> Input Signal/79(VINP_RrRegenAvailTq_Nm)
  [VINP_FrEDURealTMTqNidec_Nm] -> Input Signal/80(VINP_FrEDURealTMTqNidec_Nm)
  [VINP_FrEDURealTMTq_Nm] -> Input Signal/81(VINP_FrEDURealTMTq_Nm)
  [VINP_RrEDURealTMTqNidec_Nm] -> Input Signal/82(VINP_RrEDURealTMTqNidec_Nm)
  [VINP_RrEDURealTMTq_Nm] -> Input Signal/83(VINP_RrEDURealTMTq_Nm)
  [VINP_FrMotorAvailTqNidec_Nm] -> Input Signal/84(VINP_FrMotorAvailTqNidec_Nm)
  [VINP_FrMotorAvailTq_Nm] -> Input Signal/85(VINP_FrMotorAvailTq_Nm)
  [VINP_RrMotorAvailTqNidec_Nm] -> Input Signal/86(VINP_RrMotorAvailTqNidec_Nm)
  [VINP_RrMotorAvailTq_Nm] -> Input Signal/87(VINP_RrMotorAvailTq_Nm)
  [VINP_MCUWarnFNidec_enum] -> Input Signal/88(VINP_MCUWarnFNidec_enum)
  [VINP_MCUWarnF_enum] -> Input Signal/89(VINP_MCUWarnF_enum)
  [VINP_MCUWarnRNidec_enum] -> Input Signal/90(VINP_MCUWarnRNidec_enum)
  [VINP_MCUWarnR_enum] -> Input Signal/91(VINP_MCUWarnR_enum)
  [VINP_FrMCUDCBusVoltNidec_V] -> Input Signal/92(VINP_FrMCUDCBusVoltNidec_V)
  [VINP_FrMCUDCBusVolt_V] -> Input Signal/93(VINP_FrMCUDCBusVolt_V)
  [VINP_RrMCUDCBusVoltNidec_V] -> Input Signal/94(VINP_RrMCUDCBusVoltNidec_V)
  [VINP_RrMCUDCBusVolt_V] -> Input Signal/95(VINP_RrMCUDCBusVolt_V)
  [VINP_FrMCUTempNidec_C] -> Input Signal/96(VINP_FrMCUTempNidec_C)
  [VINP_FrMCUTemp_C] -> Input Signal/97(VINP_FrMCUTemp_C)
  [VINP_FrTMTempNidec_C] -> Input Signal/98(VINP_FrTMTempNidec_C)
  [VINP_FrTMTemp_C] -> Input Signal/99(VINP_FrTMTemp_C)
  [VINP_RrMCUTempNidec_C] -> Input Signal/100(VINP_RrMCUTempNidec_C)
  [VINP_RrMCUTemp_C] -> Input Signal/101(VINP_RrMCUTemp_C)
  [VINP_RrTMTempNidec_C] -> Input Signal/102(VINP_RrTMTempNidec_C)
  [VINP_RrTMTemp_C] -> Input Signal/103(VINP_RrTMTemp_C)
  [VINP_SWCResUpSta_flg] -> Input Signal/104(VINP_SWCResUpSta_flg)
  [VINP_SWCSetdownSta_flg] -> Input Signal/105(VINP_SWCSetdownSta_flg)
  [VINP_SWCACCSta_flg] -> Input Signal/106(VINP_SWCACCSta_flg)
  [VINP_SWCCANCELSta_flg] -> Input Signal/107(VINP_SWCCANCELSta_flg)
  [VINP_SWC2LScrollUpSta_flg] -> Input Signal/108(VINP_SWC2LScrollUpSta_flg)
  [VINP_SWC2LScrollDownSta_flg] -> Input Signal/109(VINP_SWC2LScrollDownSta_flg)
  [VINP_SWC2LScrollPressSta_flg] -> Input Signal/110(VINP_SWC2LScrollPressSta_flg)
  [VINP_SWC2LADASSta_flg] -> Input Signal/111(VINP_SWC2LADASSta_flg)
  [VINP_SWC2RScrollPressSta_flg] -> Input Signal/112(VINP_SWC2RScrollPressSta_flg)
  [VINP_SWC2RScrollUpSta_flg] -> Input Signal/113(VINP_SWC2RScrollUpSta_flg)
  [VINP_SWC2RScrollDownSta_flg] -> Input Signal/114(VINP_SWC2RScrollDownSta_flg)
  [VINP_SWC2LDriveModeSta_flg] -> Input Signal/115(VINP_SWC2LDriveModeSta_flg)
  [VINP_SWC2RRightSta_flg] -> Input Signal/116(VINP_SWC2RRightSta_flg)
  [VINP_SWC2RLeftSta_flg] -> Input Signal/117(VINP_SWC2RLeftSta_flg)
  [VINP_SWCRegenUp_flg] -> Input Signal/118(VINP_SWCRegenUp_flg)
  [VINP_SWC2RCustomizeSta_flg] -> Input Signal/119(VINP_SWC2RCustomizeSta_flg)
  [VINP_SWC2LRegenUpSta_flg] -> Input Signal/120(VINP_SWC2LRegenUpSta_flg)
  [VINP_SWC2RRegenDownSta_flg] -> Input Signal/121(VINP_SWC2RRegenDownSta_flg)
  [VINP_SWCRegenDown_flg] -> Input Signal/122(VINP_SWCRegenDown_flg)
  [VVMC_ADASForceIdle_flg] -> Input Signal/123(VVMC_ADASForceIdle_flg)
  [VVMC_ACCRequiredAccel_mps2] -> Input Signal/124(VVMC_ACCRequiredAccel_mps2)
  [VVMC_ACCVehHoldReq_flg] -> Input Signal/125(VVMC_ACCVehHoldReq_flg)
  [VVMC_ADASActive_flg] -> Input Signal/126(VVMC_ADASActive_flg)
  [VVMC_ADASWhlTqReq_Nm] -> Input Signal/127(VVMC_ADASWhlTqReq_Nm)
  [VVMC_CruzActive_flg] -> Input Signal/128(VVMC_CruzActive_flg)
  [VVMC_CruzWhlTqReq_Nm] -> Input Signal/129(VVMC_CruzWhlTqReq_Nm)
  [VVMC_MSAActive_flg] -> Input Signal/130(VVMC_MSAActive_flg)
  [VVMC_MSAWhlTqReq_Nm] -> Input Signal/131(VVMC_MSAWhlTqReq_Nm)
  [VVMC_APSActive_flg] -> Input Signal/132(VVMC_APSActive_flg)
  [VVMC_APSSpeedCMD_kph] -> Input Signal/133(VVMC_APSSpeedCMD_kph)
  [VVMC_APSShiftPosnReq_enum] -> Input Signal/134(VVMC_APSShiftPosnReq_enum)
  [VVMC_ACCPedalOvrd_flg] -> Input Signal/135(VVMC_ACCPedalOvrd_flg)
  [VVMC_LongAcc_Gps] -> Input Signal/136(VVMC_LongAcc_Gps)
  [VVMC_ActMaxSlideRate_pct] -> Input Signal/137(VVMC_ActMaxSlideRate_pct)
  [VVMC_EstSlope_Deg] -> Input Signal/138(VVMC_EstSlope_Deg)
  [VVMC_APSReq_enum] -> Input Signal/139(VVMC_APSReq_enum)
  [VVMC_RWDRDCActive_enum] -> Input Signal/140(VVMC_RWDRDCActive_enum)
  [VVMC_ActLRSlideRate_pct] -> Input Signal/141(VVMC_ActLRSlideRate_pct)
  [VVMC_ActRRSlideRate_pct] -> Input Signal/142(VVMC_ActRRSlideRate_pct)
  [VVMC_ActStESCYaw_Dps] -> Input Signal/143(VVMC_ActStESCYaw_Dps)
  [VVMC_CCCtrlSta_enum] -> Input Signal/144(VVMC_CCCtrlSta_enum)
  [VVMC_MSACtrlSta_enum] -> Input Signal/145(VVMC_MSACtrlSta_enum)
  [VVMC_LVDAACCStatusInformation_flg] -> Input Signal/146(VVMC_LVDAACCStatusInformation_flg)
  [VVMC_ACCObjDist_m] -> Input Signal/147(VVMC_ACCObjDist_m)
  [VVMC_MeterIndSpeed_raw32] -> Input Signal/148(VVMC_MeterIndSpeed_raw32)
  [VVMC_RearTqRatio_rat] -> Input Signal/149(VVMC_RearTqRatio_rat)
  [VVMC_CalibratedGyroY_Dps] -> Input Signal/150(VVMC_CalibratedGyroY_Dps)
  [VVMC_CAASActive_flg] -> Input Signal/151(VVMC_CAASActive_flg)
  [VVMC_SetACCDisableAPS_flg] -> Input Signal/152(VVMC_SetACCDisableAPS_flg)
  [VINP_BrakeSWGPIO_flg] -> Input Signal/155(VINP_BrakeSWGPIO_flg)
  [VINP_CrashSignalGPIO_flg] -> Input Signal/156(VINP_CrashSignalGPIO_flg)
  [VINP_DrDoorSW_flg] -> Input Signal/157(VINP_DrDoorSW_flg)
  [VINP_SeatSW_flg] -> Input Signal/158(VINP_SeatSW_flg)
  [VINP_HoodSW_flg] -> Input Signal/159(VINP_HoodSW_flg)
  [VINP_TailgateSW_flg] -> Input Signal/160(VINP_TailgateSW_flg)
  [VINP_PsDoorSW_flg] -> Input Signal/161(VINP_PsDoorSW_flg)
  [VINP_RRDoorSW_flg] -> Input Signal/162(VINP_RRDoorSW_flg)
  [VINP_RLDoorSW_flg] -> Input Signal/163(VINP_RLDoorSW_flg)
  [VBCM_BrakeLamp_flg] -> Input Signal/164(VBCM_BrakeLamp_flg)
  [VBCM_UserNow_enum] -> Input Signal/165(VBCM_UserNow_enum)
  [VINP_ADASISASta_enum] -> Input Signal/166(VINP_ADASISASta_enum)
  [VINP_ADASVehSpdLim_enum] -> Input Signal/167(VINP_ADASVehSpdLim_enum)
  [VINP_ADASACCSta_enum] -> Input Signal/168(VINP_ADASACCSta_enum)
  [VINP_ADASSLIFSpdLim_enum] -> Input Signal/169(VINP_ADASSLIFSpdLim_enum)
  [VINP_ADASAEBSta_enum] -> Input Signal/170(VINP_ADASAEBSta_enum)
  [VINP_FlashRegenMode_enum] -> Input Signal/172(VINP_FlashRegenMode_enum)
  [VINP_VehicleType_enum] -> Input Signal/173(VINP_VehicleType_enum)
  [VINP_SWCType_enum] -> Input Signal/174(VINP_SWCType_enum)
  [VINP_CAASSta_enum] -> Input Signal/175(VINP_CAASSta_enum)
  [VINP_APSStaSystem_enum] -> Input Signal/176(VINP_APSStaSystem_enum)
  [VDDM_VCURAPSErrLv2_flg] -> Input Signal/177(VDDM_VCURAPSErrLv2_flg)
  [VDDM_VCURAPSErrLv3_flg] -> Input Signal/178(VDDM_VCURAPSErrLv3_flg)
  [VDDM_EPBSigErrCFS_flg] -> Input Signal/179(VDDM_EPBSigErrCFS_flg)
  [VDDM_EPB1Err_flg] -> Input Signal/180(VDDM_EPB1Err_flg)
  [VDDM_ESC1Err_flg] -> Input Signal/181(VDDM_ESC1Err_flg)
  [VDDM_ESC5Err_flg] -> Input Signal/182(VDDM_ESC5Err_flg)
  [VDDM_LimpHomeAct_flg] -> Input Signal/183(VDDM_LimpHomeAct_flg)
  [VDDM_VehMalfunLevel_enum] -> Input Signal/184(VDDM_VehMalfunLevel_enum)
  [VDDM_Shifter1Err_flg] -> Input Signal/185(VDDM_Shifter1Err_flg)
  [VDDM_ShifterSigErrCFS_flg] -> Input Signal/186(VDDM_ShifterSigErrCFS_flg)
  [VDDM_MCUF1Err_flg] -> Input Signal/187(VDDM_MCUF1Err_flg)
  [VDDM_MCUR1Err_flg] -> Input Signal/188(VDDM_MCUR1Err_flg)
  [VDDM_RegenErrCFS_flg] -> Input Signal/189(VDDM_RegenErrCFS_flg)
  [VDDM_4D2CErr_flg] -> Input Signal/190(VDDM_4D2CErr_flg)
  [VINP_PBWMotorPos_enum] -> Input Signal/191(VINP_PBWMotorPos_enum)
  [VBCM_RegenModeUserSetting_enum] -> Input Signal/192(VBCM_RegenModeUserSetting_enum)
  [VINP_IVIEscapeModeCmd_flg] -> Input Signal/193(VINP_IVIEscapeModeCmd_flg)
  Input Signal/1(BSCPIn_outputs) -> BSCPIn_outputs/1
  [VINP_BrkSwV_flg] -> Invalid Condition/1(VINP_BrkSwV_flg)
  [VINP_BrkSwSta_flg] -> Input Signal/10(VINP_BrkSwSta_flg)
  [VINP_BrkSwV_flg] -> Input Signal/11(VINP_BrkSwV_flg)
  [VINP_BrkPedalPosSta_flg] -> Invalid Condition/2(VINP_BrkPedalPosSta_flg)
  [VINP_ShifterHandleCmd_enum] -> Invalid Condition/3(VINP_ShifterHandleCmd_enum)
  [VDDM_Shifter1Err_flg] -> Invalid Condition/4(VDDM_Shifter1Err_flg)
  [BInInvalid_outputs] -> Input Signal/1(BInInvalid_outputs)
  Invalid Condition/1(BInInvalid_outputs) -> [BInInvalid_outputs]
  Bus Selector5/31 -> [VVMC_CCPedalOvrd_flg]  "<VVMC_CCPedalOvrd_flg>"
  [VVMC_CCPedalOvrd_flg] -> Input Signal/153(VVMC_CCPedalOvrd_flg)
  Bus Selector5/32 -> [VVMC_MSAWhlTqActive_flg]  "<VVMC_MSAWhlTqActive_flg>"
  [VVMC_MSAWhlTqActive_flg] -> Input Signal/154(VVMC_MSAWhlTqActive_flg)
  Bus Selector9/6 -> [VINP_ACCVehHoldReq_flg]  "<VINP_ACCVehHoldReq_flg>"
  [VINP_ACCVehHoldReq_flg] -> Input Signal/171(VINP_ACCVehHoldReq_flg)
  Constant3/1 -> [VINP_DIDExhibitMode_enum]  "VTQD_DIDExhibitMode_enum"
  [VINP_DIDExhibitMode_enum] -> Input Signal/194(VINP_DIDExhibitMode_enum)
  Bus Selector11/4 -> [VINP_DIDGetDynoMode_flg]  "<VINP_DIDGetDynoMode_flg>"
  [VINP_DIDGetDynoMode_flg] -> Input Signal/195(VINP_DIDGetDynoMode_flg)
  Bus Selector11/5 -> [VINP_CAN1BusOff_flg]  "<VINP_CAN1BusOff_flg>"
  Bus Selector11/6 -> [VINP_CAN1BusError_flg]  "<VINP_CAN1BusError_flg>"
  Bus Selector11/7 -> [VINP_CAN2BusOff_flg]  "<VINP_CAN2BusOff_flg>"
  Bus Selector11/8 -> [VINP_CAN2BusError_flg]  "<VINP_CAN2BusError_flg>"
  Constant12/1 -> [VINP_DIDNVHPedalLim_flg]  "VINP_DIDNVHPedalLim_flg"
  [VINP_CAN1BusOff_flg] -> Input Signal/196(VINP_CAN1BusOff_flg)
  [VINP_CAN1BusError_flg] -> Input Signal/197(VINP_CAN1BusError_flg)
  [VINP_CAN2BusOff_flg] -> Input Signal/198(VINP_CAN2BusOff_flg)
  [VINP_CAN2BusError_flg] -> Input Signal/199(VINP_CAN2BusError_flg)
  [VINP_DIDNVHPedalLim_flg] -> Input Signal/200(VINP_DIDNVHPedalLim_flg)
  Ground/1 -> [VINP_SCPSystemMode_enum]
  [VINP_SCPSystemMode_enum] -> Input Signal/201(VINP_SCPSystemMode_enum)
  Ground1/1 -> [VDDM_EPB1NoComCFS_flg]
  Ground2/1 -> [VDDM_EPB1RCErrCFS_flg]
  Ground3/1 -> [VDDM_EPB1CSErrCFS_flg]
  [VDDM_EPB1NoComCFS_flg] -> Input Signal/202(VDDM_EPB1NoComCFS_flg)
  [VDDM_EPB1RCErrCFS_flg] -> Input Signal/203(VDDM_EPB1RCErrCFS_flg)
  [VDDM_EPB1CSErrCFS_flg] -> Input Signal/204(VDDM_EPB1CSErrCFS_flg)
  Bus Selector7/4 -> [VPMM_DrSeatSta_enum]  "<VPMM_DrSeatSta_enum>"
  [VPMM_DrSeatSta_enum] -> Input Signal/8(VPMM_DrSeatSta_enum)
  Bus Selector2/37 -> [VINP_MCPressure_bar]  "<VINP_MCPressure_bar>"
  [VINP_MCPressure_bar] -> Input Signal/45(VINP_MCPressure_bar)
  Ground4/1 -> [VBCM_CTDCtrl_enum]
  Ground5/1 -> [VINP_FlashCrashDetd_flg]
  Ground6/1 -> [VINP_FlashCrashUnlockReq_flg]
  Ground7/1 -> [VBCM_CrashUnlkSuccess_flg]
  [VBCM_CTDCtrl_enum] -> Input Signal/205(VBCM_CTDCtrl_enum)
  [VINP_FlashCrashDetd_flg] -> Input Signal/206(VINP_FlashCrashDetd_flg)
  [VINP_FlashCrashUnlockReq_flg] -> Input Signal/207(VINP_FlashCrashUnlockReq_flg)
  [VBCM_CrashUnlkSuccess_flg] -> Input Signal/208(VBCM_CrashUnlkSuccess_flg)
